simulink model "TesteDegrauMinQuadSimulinkY"  (R2015a)
settings: Solver=ode45  StartTime=0.0  StopTime=51  RelTol=1e-3
values from neighbouring files (symbols this model uses):
  T = 0.04    [Minimos_Quadrados.m]    (also in TesteDegrauMinQuad.m = 0.03)
  tf_digital_dnY = MinimosQuadrados(N, y, u, T, ordem)    [Minimos_Quadrados.m]
  tf_digital_dpY = MinimosQuadrados(N, y, u, T, ordem)    [Minimos_Quadrados.m]
  tf_digital_wnY = MinimosQuadrados(N, y, u, T, ordem)    [Minimos_Quadrados.m]
settings Model: Creator=Lucas  LastModifiedBy=Lucas

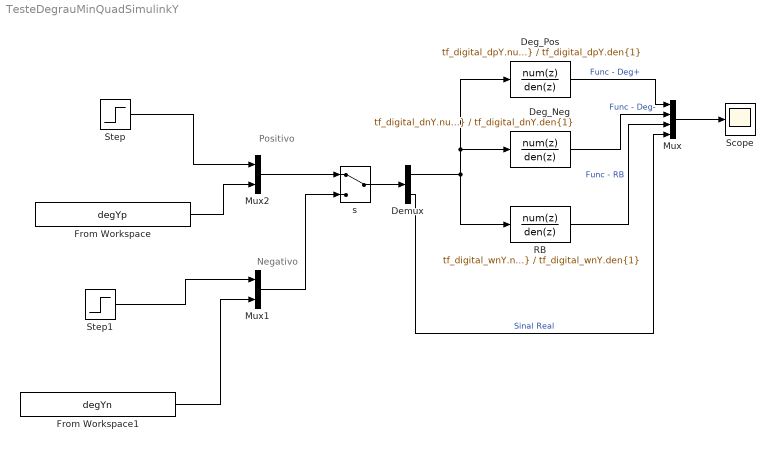
== system TesteDegrauMinQuadSimulinkY ==
  note: Positivo
  note: Negativo
  Deg_Neg : DiscreteTransferFcn  Numerator=tf_digital_dnY.num{1}  Denominator=tf_digital_dnY.den{1}  SampleTime=T
  Deg_Pos : DiscreteTransferFcn  Numerator=tf_digital_dpY.num{1}  Denominator=tf_digital_dpY.den{1}  SampleTime=T
  Demux : Demux  Outputs=2
  From Workspace : FromWorkspace  VariableName=degYp  SampleTime=T
  From Workspace1 : FromWorkspace  VariableName=degYn  SampleTime=T
  Mux : Mux
  Mux1 : Mux  Inputs=2
  Mux2 : Mux  Inputs=2
  RB : DiscreteTransferFcn  Numerator=tf_digital_wnY.num{1}  Denominator=tf_digital_wnY.den{1}  SampleTime=T
  Scope : Scope
      settings: ShowLegends=on
  Step : Step  Time=11  After=10  SampleTime=T
  Step1 : Step  Time=11  After=-10  SampleTime=T
  s : ManualSwitch
  wires:
  Deg_Pos/1 -> Mux/1  "Func - Deg+"
  Mux/1 -> Scope/1
  Deg_Neg/1 -> Mux/2  "Func - Deg-"
  s/1 -> Demux/1
  Demux/2 -> Mux/4  "Sinal Real"
  Demux/1 -> Deg_Pos/1, Deg_Neg/1, RB/1
  From Workspace/1 -> Mux2/2
  Step/1 -> Mux2/1
  From Workspace1/1 -> Mux1/2
  Step1/1 -> Mux1/1
  Mux1/1 -> s/2
  Mux2/1 -> s/1
  RB/1 -> Mux/3  "Func - RB"
